simulink model "model_03"  (R2021b)
settings: Solver=ode45  StartTime=0.0  StopTime=10  RelTol=1e-3
settings Model: Creator=jimd  LastModifiedBy=jimd

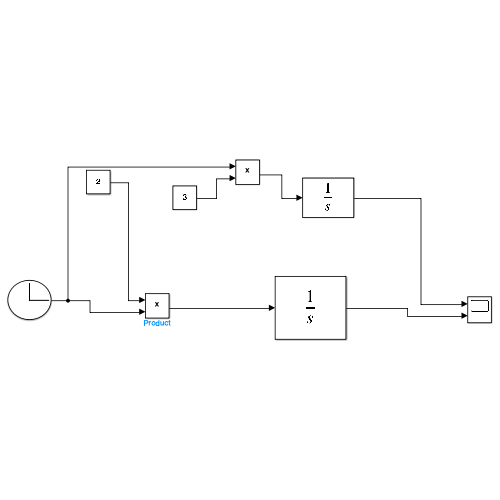
[thumbnail: Simulink's stored preview of the top-level diagram]
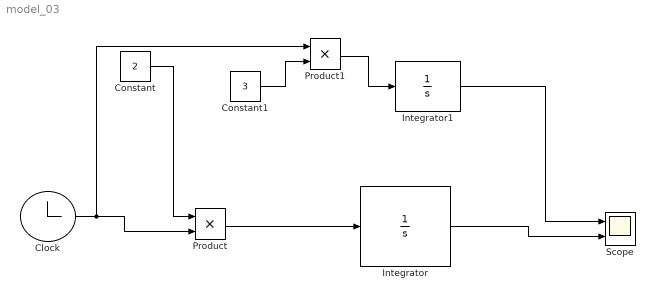
== system model_03 ==
  Clock : Clock
  Constant : Constant  Value=2
  Constant1 : Constant  Value=3
  Integrator : Integrator
  Integrator1 : Integrator
  Product : Product
  Product1 : Product
  Scope : Scope  NumInputPorts=2
  wires:
  Constant/1 -> Product/1
  Clock/1 -> Product1/1, Product/2
  Product/1 -> Integrator/1
  Integrator/1 -> Scope/2
  Constant1/1 -> Product1/2
  Product1/1 -> Integrator1/1
  Integrator1/1 -> Scope/1
